simulink model "testCG"  (R2025b)
settings: Solver=FixedStepDiscrete  StartTime=0.0  StopTime=10.0  FixedStep=0.1  RelTol=1e-3
values from neighbouring files (symbols this model uses):
  A = 0.95    [myDD.sldd]    (also in myDDFinal.sldd = 0.95
  B = 0.25    [myDD.sldd]    (also in myDDFinal.sldd = 0.25
  C = 0.2    [myDD.sldd]    (also in myDDFinal.sldd = 0.2
  D = 0.0    [myDD.sldd]    (also in myDDFinal.sldd = 0.0
settings Model: DataDictionary=myDD.sldd  Creator=grouleau  LastModifiedBy=guirl
settings DataIOCC: ExternalInput=[0, 1]  LoadExternalInput=on  SaveFormat=Array
settings OptimizationCC: EnhancedBackFolding=on  PassReuseOutputArgsAs=Individual arguments  ZeroExternalMemoryAtStartup=off  ZeroInternalMemoryAtStartup=off  OptimizeBlockOrder=speed  DifferentSizesBufferReuse=on  OptimizationCustomize=off  EfficientTunableParamExpr=on
settings DebuggingCC: ParameterTunabilityLossMsg=error
settings SFSimCC: MATLABDynamicMemAlloc=off
settings RTWCC: SystemTargetFile=ert.tlc  GenCodeOnly=on  TemplateMakefile=ert_default_tmf  RTWVerbose=off  Description=Embedded Coder
settings CodeAppCC: ForceParamTrailComments=on  IgnoreCustomStorageClasses=off  OperatorAnnotations=on  SimulinkDataObjDesc=on  SFDataObjDesc=on  InsertBlockDesc=on
settings ERTTargetCC: InlinedParameterPlacement=Hierarchical  ERTCustomFileTemplate=example_file_process.tlc  TargetLangStandard=C99 (ISO)  GenerateSampleERTMain=on

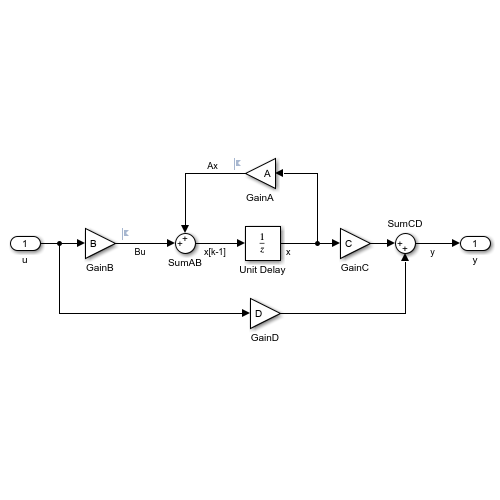
[thumbnail: Simulink's stored preview of the top-level diagram]
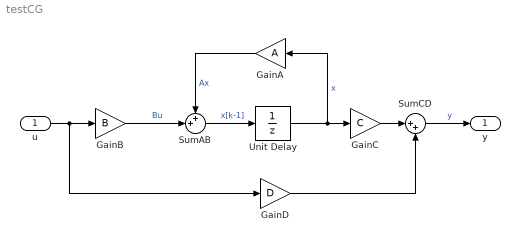
== system testCG ==
  u : Inport
  GainA : Gain  Gain=A
  GainB : Gain  Gain=B
  GainC : Gain  Gain=C
  GainD : Gain  Gain=D
  SumAB : Sum  Inputs=++|
  SumCD : Sum  Inputs=|++
  Unit Delay : UnitDelay  SampleTime=-1  HasFrameUpgradeWarning=on
  y : Outport
  wires:
  Unit Delay/1 -> GainA/1, GainC/1  "x"
  u/1 -> GainD/1, GainB/1
  SumCD/1 -> y/1  "y"
  SumAB/1 -> Unit Delay/1  "x[k-1]"
  GainB/1 -> SumAB/2  "Bu"
  GainA/1 -> SumAB/1  "Ax"
  GainC/1 -> SumCD/1
  GainD/1 -> SumCD/2
